simulink model "LR5_graph_1"  (R2018a)
settings: Solver=ode45  StartTime=0.0  StopTime=20  RelTol=1e-3  EnableMultiTasking=on
settings Model: Creator=stud507ikt  LastModifiedBy=Asus
settings DataIOCC: LimitDataPoints=on  SaveFormat=Array
settings OptimizationCC: LifeSpan=inf
settings DebuggingCC: SolverPrmCheckMsg=warning  SFUnexpectedBacktrackingDiag=warning  SFNoUnconditionalDefaultTransitionDiag=warning  SFExecutionAtInitializationDiag=none
settings HardwareCC: ProdBitPerPointer=32  ProdBitPerSizeT=32  ProdBitPerPtrDiffT=32  ProdLargestAtomicFloat=None  ProdIntDivRoundTo=Undefined  ProdEndianess=Unspecified  ProdWordSize=32  ProdHWDeviceType=32-bit Generic
settings ModelReferenceCC: PropagateSignalLabelsOutOfModel=off
settings CodeAppCC: StateflowObjectComments=on
settings GRTTargetCC: TargetLangStandard=C89/C90 (ANSI)  GeneratePreprocessorConditionals=Disable all
settings ConfigComp: CovMetricSettings=dw  CovHtmlReporting=on  CovSaveCumulativeToWorkspaceVar=on  CovSaveSingleToWorkspaceVar=on  CovExternalEMLEnable=off  CovSFcnEnable=off

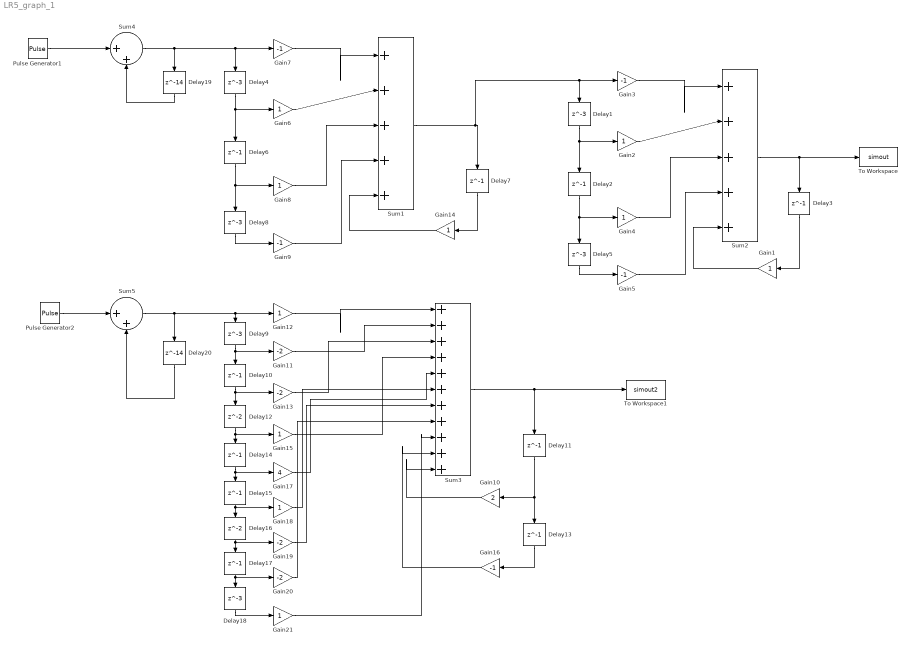
== system LR5_graph_1 ==
  Delay{1,4..5,8..9,18} (6 alike) : Delay  DelayLength=3  InitialCondition=0  InputProcessing=Inherited
  Delay{2..3,6..7,10..11,13..15,17} (10 alike) : Delay  DelayLength=1  InitialCondition=0  InputProcessing=Inherited
  Delay12 : Delay  InitialCondition=0  InputProcessing=Inherited
  Delay16 : Delay  InitialCondition=0  InputProcessing=Inherited
  Delay19 : Delay  DelayLength=14  InitialCondition=0  InputProcessing=Inherited
  Delay20 : Delay  DelayLength=14  InitialCondition=0  InputProcessing=Inherited
  Gain{1..2,4,6,8,12,14..15,18,21} (10 alike) : Gain
  Gain10 : Gain  Gain=2
  Gain{11,13,19..20} (4 alike) : Gain  Gain=-2
  Gain{3,5,7,9,16} (5 alike) : Gain  Gain=-1
  Gain17 : Gain  Gain=4
  Pulse Generator1 : DiscretePulseGenerator  Period=10000
  Pulse Generator2 : DiscretePulseGenerator  Period=10000
  Sum1 : Sum  Inputs=|+++++
  Sum2 : Sum  Inputs=|+++++
  Sum3 : Sum  Inputs=|+++++++++++
  Sum4 : Sum  Inputs=|++
  Sum5 : Sum  Inputs=|++
  To Workspace : ToWorkspace  VariableName=simout  SampleTime=-1
  To Workspace1 : ToWorkspace  VariableName=simout2  SampleTime=-1
  wires:
  Gain6/1 -> Sum1/2
  Gain7/1 -> Sum1/1
  Gain8/1 -> Sum1/3
  Delay6/1 -> Delay8/1, Gain8/1
  Delay8/1 -> Gain9/1
  Gain9/1 -> Sum1/4
  Pulse Generator1/1 -> Sum4/1
  Delay7/1 -> Gain14/1
  Delay4/1 -> Delay6/1, Gain6/1
  Gain14/1 -> Sum1/5
  Gain2/1 -> Sum2/2
  Gain3/1 -> Sum2/1
  Gain4/1 -> Sum2/3
  Delay2/1 -> Delay5/1, Gain4/1
  Delay5/1 -> Gain5/1
  Gain5/1 -> Sum2/4
  Sum1/1 -> Gain3/1, Delay1/1, Delay7/1
  Delay3/1 -> Gain1/1
  Delay1/1 -> Delay2/1, Gain2/1
  Sum2/1 -> To Workspace/1, Delay3/1
  Gain1/1 -> Sum2/5
  Gain12/1 -> Sum3/1
  Delay11/1 -> Delay13/1, Gain10/1
  Gain10/1 -> Sum3/11
  Delay13/1 -> Gain16/1
  Gain16/1 -> Sum3/10
  Sum3/1 -> Delay11/1, To Workspace1/1
  Gain11/1 -> Sum3/2
  Delay9/1 -> Delay10/1, Gain11/1
  Delay10/1 -> Delay12/1, Gain13/1
  Gain13/1 -> Sum3/3
  Delay12/1 -> Delay14/1, Gain15/1
  Gain15/1 -> Sum3/4
  Delay14/1 -> Gain17/1, Delay15/1
  Gain17/1 -> Sum3/5
  Gain18/1 -> Sum3/6
  Gain19/1 -> Sum3/7
  Delay16/1 -> Delay17/1, Gain19/1
  Delay15/1 -> Delay16/1, Gain18/1
  Delay17/1 -> Delay18/1, Gain20/1
  Gain20/1 -> Sum3/8
  Delay18/1 -> Gain21/1
  Gain21/1 -> Sum3/9
  Sum4/1 -> Delay19/1, Delay4/1, Gain7/1
  Delay19/1 -> Sum4/2
  Delay20/1 -> Sum5/2
  Sum5/1 -> Delay9/1, Gain12/1, Delay20/1
  Pulse Generator2/1 -> Sum5/1
